simulink model "SCARA_Robot"  (R2018b)
settings: Solver=FixedStepAuto  StartTime=0.0  StopTime=5  FixedStep=0.001  MaxStep=0.001  MinStep=0.0001  RelTol=1e-3
model workspace: external: MATLAB File G:\MATLAB\SCARA\SCARA_Robot_DataFile.m (data not in the file)
values from neighbouring files (symbols this model uses):
  Ball = struct    [SCARA_Robot_DataFile.m]
  Plane = struct    [SCARA_Robot_DataFile.m]
  smiData = struct    [SCARA_Robot_DataFile.m]
undefined symbols (not defined in the file or in its folder): sigbuilder_block, X, Y, Z
libraries: sm_lib x160, nesl_utility x83, robotmaniplib x17, Contact_Forces_Lib x6, Parts_Lib x4, simulink x1
(part 1 of 4)
settings Model: Creator=wqq  LastModifiedBy=wqq
settings SolverCC: InitialStep=0.0001

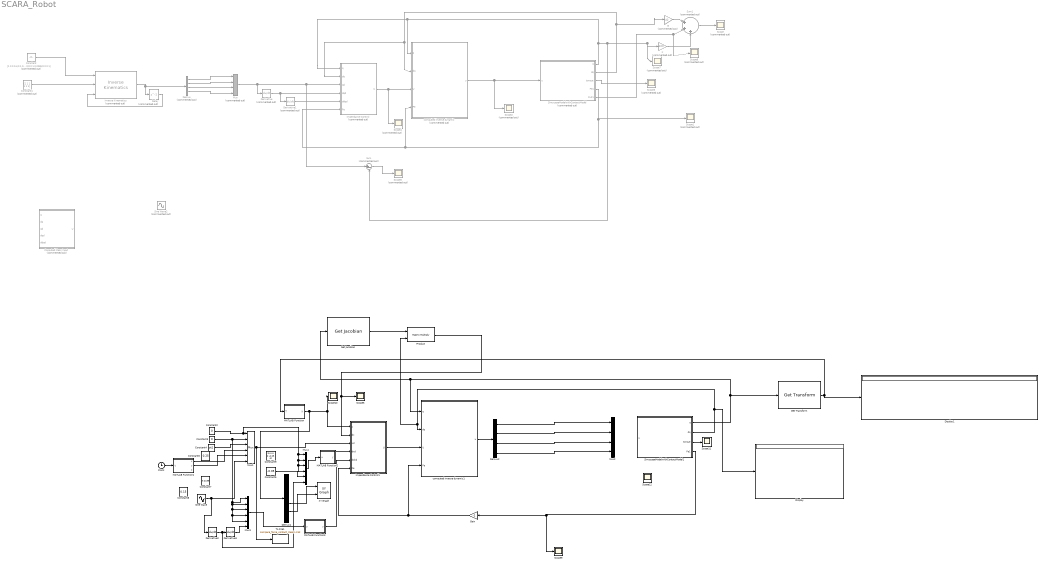
== system SCARA_Robot ==
  B : Gain  Commented=on  Gain=40
  Clock : Clock
  Conputed Mass Input : Subsystem  Commented=on
  Constant : Constant  Commented=on  Value=[1 0 0 0.4;0 1 0 0;0 0 1 0.2235;0 0 0 1]  VectorParams1D=off
  Constant1 : Constant  Commented=on  Value=[1 1 1 1 1 1]
  Constant2 : Constant  Value=0
  Constant3 : Constant  Value=0
  Constant4 : Constant  Value=pi/2
  Constant5 : Constant  Value=-0.05  VectorParams1D=off
  Constant6 : Constant  Value=0.25
  Constant7 : Constant  Value=0.2235
  Constant8 : Constant  Value=0.15
  Constant9 : Constant  Value=[0 0 0 0 -0.05 0]  VectorParams1D=off
  Delay : Delay  Commented=on  DelayLength=1  InitialCondition=[0;0;0;0]
  Demux : Demux  Commented=on
  Demux1 : Demux  Outputs=6
  Demux2 : Demux
  Derivative : Derivative  Commented=on
  Derivative1 : Derivative  Commented=on
  Derivative2 : Derivative
  Derivative3 : Derivative
  Display : Display
  Display1 : Display
  Gain : Gain  Gain=-1
  Get Jacobian : robotmaniplib/Get Jacobian  RigidBodyTree=SCARA_Robot  EndEffector=Body5
      settings: SourceProductName=Robotics System Toolbox
  Get Transform : robotmaniplib/Get Transform  RigidBodyTree=SCARA_Robot  SourceBody=Body5  TargetBody=Body7
      settings: SourceProductName=Robotics System Toolbox
  Impendance Control : Subsystem  Commented=on
  Impendance Control1 : Subsystem
  Inverse Kinematics : robotmaniplib/Inverse Kinematics  Commented=on  RigidBodyTree=SCARA_Robot  EndEffector=Body5  ShowInfo=off  SolverName=BFGS Gradient Projection  EnforceJointLimits=on  MaxIterations=1500  MaxTime=10  GradientTolerance=1e-7  SolutionTolerance=1e-6  StepTolerance=1e-14  ErrorChangeTolerance=1e-12  UseErrorDamping=on  DampingBias=0.0025
      settings: SourceProductName=Robotics System Toolbox
  K : Gain  Commented=on  Gain=400
  MATLAB Function : MATLAB Function  TreatAsAtomicUnit=on
  MATLAB Function1 : MATLAB Function  TreatAsAtomicUnit=on
  MATLAB Function2 : MATLAB Function  TreatAsAtomicUnit=on
  MATLAB Function3 : MATLAB Function  TreatAsAtomicUnit=on
  Mux : Mux  Commented=on
  Mux1 : Mux  Inputs=6
  Mux2 : Mux
  Mux3 : Mux  Inputs=6
  Mux4 : Mux  Inputs=6
  Product : Product  Multiplication=Matrix(*)
  Scope{,1..4,6..8} (8 alike) : Scope  Commented=on
  Scope{5,9..12} (5 alike) : Scope
  SimscapeModelwithContactModel : Subsystem  Commented=on
  SimscapeModelwithContactModel1 : Subsystem
  Sine Wave : Sin  Amplitude=0.5  Bias=0.2235  Frequency=3  SampleTime=0
  Sine Wave2 : Sin  Commented=on  Amplitude=0.5  SampleTime=0
  Sum : Sum  Commented=on  Inputs=|+-
  Sum1 : Sum  Commented=on  Inputs=|+++
  To File1 : ToFile  Filename=compare_force_contact_RealX.mat  MatrixName=RealX  SaveFormat=Timeseries
  XY Graph : simulink/Sinks/XY Graph  xmin=-0.4  xmax=0.4  ymin=-0.4  ymax=0.4  st=-1
  computed Inverse dynamic : Subsystem  Commented=on
  computed Inverse dynamic1 : Subsystem
  wires:
  computed Inverse dynamic/1(u) -> SimscapeModelwithContactModel/1(u), Scope2/1
  SimscapeModelwithContactModel/1(q) -> Scope7/1, K/1, Sum/2, computed Inverse dynamic/1(q), Impendance Control/1(q)
  SimscapeModelwithContactModel/3(torque) -> Scope3/1
  Impendance Control/1(U) -> Scope4/1, computed Inverse dynamic/3(U)
  Mux/1 -> Derivative/1, Sum/1, Impendance Control/3(qd)
  Derivative/1 -> Derivative1/1, Impendance Control/4(dqd)
  Derivative1/1 -> Impendance Control/5(ddqd)
  SimscapeModelwithContactModel/4(Fe1) -> Impendance Control/6(Fe), computed Inverse dynamic/4(Fe), Scope1/1
  Sum/1 -> Scope6/1
  SimscapeModelwithContactModel/2(dq) -> B/1, computed Inverse dynamic/2(dq), Impendance Control/2(dq)
  Sum1/1 -> Scope/1
  K/1 -> Sum1/3
  B/1 -> Sum1/1
  SimscapeModelwithContactModel/5(Out1) -> Scope8/1, Sum1/2
  Impendance Control1/1(U) -> computed Inverse dynamic1/3(U)
  SimscapeModelwithContactModel1/2(dq) -> Display/1, computed Inverse dynamic1/2(dq), Product/2
  SimscapeModelwithContactModel1/4(Fe1) -> Scope9/1, Gain/1
  Get Transform/1 -> MATLAB Function/1(T), Display1/1
  MATLAB Function/1(X) -> Demux1/1, Scope10/1, Impendance Control1/1(x)
  Inverse Kinematics/1 -> Demux/1, Delay/1
  Delay/1 -> Inverse Kinematics/3
  Constant/1 -> Inverse Kinematics/1
  Constant1/1 -> Inverse Kinematics/2
  Demux/1 -> Mux/1
  Demux/2 -> Mux/2
  Demux/3 -> Mux/3
  Demux/4 -> Mux/4
  Constant2/1 -> Mux4/1, Mux4/2, Mux4/3, Mux4/4, Mux1/1
  Constant3/1 -> Mux3/1, Mux3/2, Mux3/3, Mux3/4, Mux3/5, Mux1/2
  Constant4/1 -> Mux1/3
  Clock/1 -> MATLAB Function1/1(t)
  Get Jacobian/1 -> Product/1
  Product/1 -> Impendance Control1/2(dx), Scope5/1
  Demux1/4 -> XY Graph/1
  Demux1/5 -> XY Graph/2
  SimscapeModelwithContactModel1/1(q) -> Get Transform/1, computed Inverse dynamic1/1(q), Get Jacobian/1
  SimscapeModelwithContactModel1/3(torque) -> Scope11/1
  Gain/1 -> computed Inverse dynamic1/4(Fe), Impendance Control1/6(Fe)
  computed Inverse dynamic1/1(u) -> Demux2/1
  Sine Wave/1 -> Derivative2/1, Mux1/6
  Mux1/1 -> To File1/1, Impendance Control1/3(xd)
  Demux2/2 -> Mux2/2
  Demux2/3 -> Mux2/3
  Demux2/4 -> Mux2/4
  Demux2/1 -> Mux2/1
  MATLAB Function1/1(x) -> Mux1/4
  MATLAB Function1/2(y) -> Mux1/5
  Derivative2/1 -> Mux4/6, Derivative3/1
  Derivative3/1 -> Mux3/6
  Constant5/1 -> Mux4/5
  Mux4/1 -> MATLAB Function2/1(u)
  Mux3/1 -> MATLAB Function3/1(u)
  MATLAB Function3/1(y) -> Impendance Control1/5(ddxd)
  MATLAB Function2/1(y) -> Impendance Control1/4(dxd)

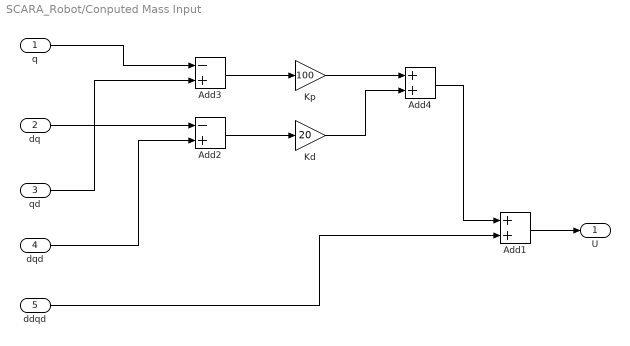
== system SCARA_Robot/Conputed Mass Input ==
  q : Inport
  dq : Inport  Port=2
  qd : Inport  Port=3
  dqd : Inport  Port=4
  ddqd : Inport  Port=5
  Add1 : Sum
  Add2 : Sum  Inputs=-+
  Add3 : Sum  Inputs=-+
  Add4 : Sum
  Kd : Gain  Gain=20
  Kp : Gain  Gain=100
  U : Outport
  wires:
  Add4/1 -> Add1/1
  Add2/1 -> Kd/1
  Kp/1 -> Add4/1
  Add3/1 -> Kp/1
  q/1 -> Add3/1
  dq/1 -> Add2/1
  dqd/1 -> Add2/2
  Add1/1 -> U/1
  Kd/1 -> Add4/2
  qd/1 -> Add3/2
  ddqd/1 -> Add1/2

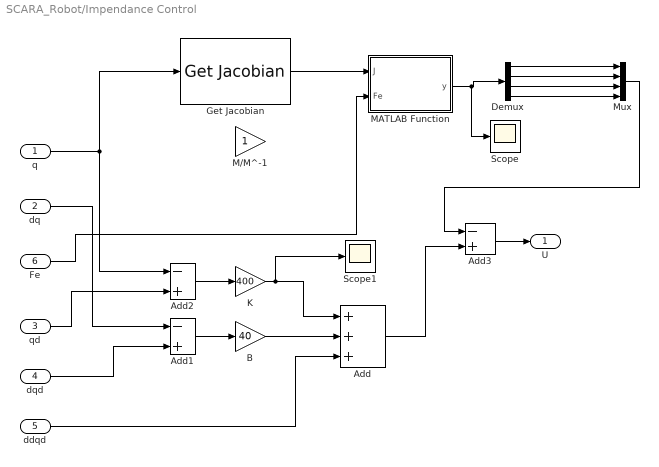
== system SCARA_Robot/Impendance Control ==
  q : Inport
  dq : Inport  Port=2
  qd : Inport  Port=3
  dqd : Inport  Port=4
  ddqd : Inport  Port=5
  Fe : Inport  Port=6
  Add : Sum  Inputs=+++
  Add1 : Sum  Inputs=-+
  Add2 : Sum  Inputs=-+
  Add3 : Sum  Inputs=-+
  B : Gain  Gain=40
  Demux : Demux
  Get Jacobian : robotmaniplib/Get Jacobian  RigidBodyTree=SCARA_Robot  EndEffector=Body5
      settings: SourceProductName=Robotics System Toolbox
  K : Gain  Gain=400
  M/M^-1 : Gain
  MATLAB Function : MATLAB Function  TreatAsAtomicUnit=on
  Mux : Mux
  Scope : Scope
  Scope1 : Scope
  U : Outport
  wires:
  ddqd/1 -> Add/3
  dqd/1 -> Add1/2
  dq/1 -> Add1/1
  Add1/1 -> B/1
  B/1 -> Add/2
  qd/1 -> Add2/2
  Add2/1 -> K/1
  K/1 -> Scope1/1, Add/1
  Add/1 -> Add3/2
  Add3/1 -> U/1
  q/1 -> Add2/1, Get Jacobian/1
  Get Jacobian/1 -> MATLAB Function/1(J)
  Fe/1 -> MATLAB Function/2(Fe)
  MATLAB Function/1(y) -> Scope/1, Demux/1
  Demux/1 -> Mux/1
  Demux/2 -> Mux/2
  Demux/3 -> Mux/3
  Demux/4 -> Mux/4
  Mux/1 -> Add3/1

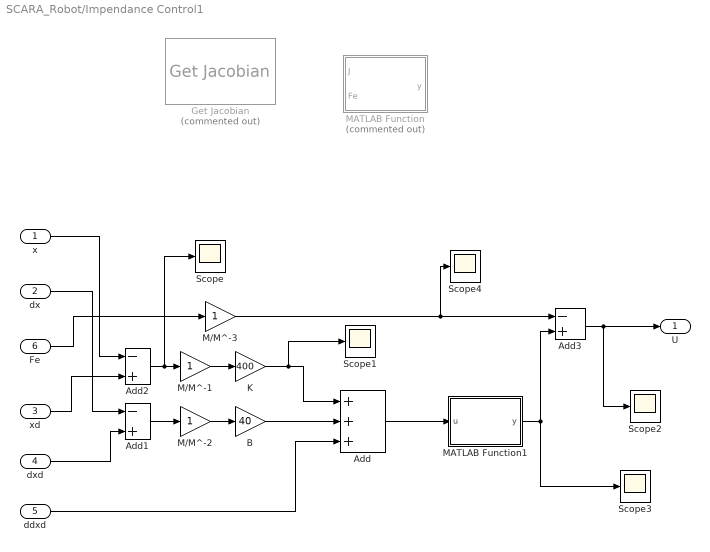
== system SCARA_Robot/Impendance Control1 ==
  x : Inport
  dx : Inport  Port=2
  xd : Inport  Port=3
  dxd : Inport  Port=4
  ddxd : Inport  Port=5
  Fe : Inport  Port=6
  Add : Sum  Inputs=+++
  Add1 : Sum  Inputs=-+
  Add2 : Sum  Inputs=-+
  Add3 : Sum  Inputs=-+
  B : Gain  Gain=40
  Get Jacobian : robotmaniplib/Get Jacobian  Commented=on  RigidBodyTree=SCARA_Robot  EndEffector=Body5
      settings: SourceProductName=Robotics System Toolbox
  K : Gain  Gain=400
  M/M^-1 : Gain
  M/M^-2 : Gain
  M/M^-3 : Gain
  MATLAB Function : MATLAB Function  Commented=on  TreatAsAtomicUnit=on
  MATLAB Function1 : MATLAB Function  TreatAsAtomicUnit=on
  Scope{,1..4} (5 alike) : Scope
  U : Outport
  wires:
  ddxd/1 -> Add/3
  dxd/1 -> Add1/2
  dx/1 -> Add1/1
  Add1/1 -> M/M^-2/1
  B/1 -> Add/2
  xd/1 -> Add2/2
  Add2/1 -> Scope/1, M/M^-1/1
  K/1 -> Scope1/1, Add/1
  Add/1 -> MATLAB Function1/1(u)
  x/1 -> Add2/1
  Fe/1 -> M/M^-3/1
  M/M^-1/1 -> K/1
  M/M^-2/1 -> B/1
  M/M^-3/1 -> Scope4/1, Add3/1
  MATLAB Function1/1(y) -> Add3/2, Scope3/1
  Add3/1 -> Scope2/1, U/1

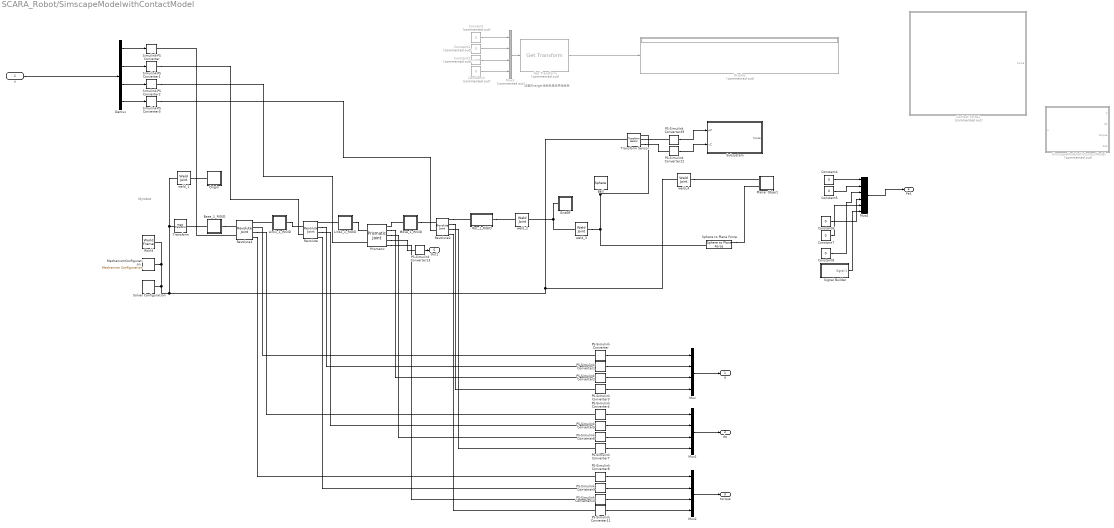
== system SCARA_Robot/SimscapeModelwithContactModel ==
  note: 这里的target坐标系是世界坐标系
  note: Myrobot
  u : Inport
  Ball : Parts_Lib/Sphere  Tag=CustomStyle  sph_radius=Ball.radius  sph_density=Ball.density  sph_color=red  sph_opacity=1  mark_type=Rings on center planes  arc_width=[40 50]  arc_angle=60  ring_width=5  ring_irad=0.95  mark_color=axes  mark_opacity_x=1  mark_opacity_y=1  mark_opacity_z=1  mark_opacity=1  ring_opacity=0  arc_opacity=0  arc_extr_data=0
  Base_1_RIGID : Subsystem
  Constant : Constant  Commented=on  Value=0
  Constant1 : Constant  Commented=on  Value=0
  Constant2 : Constant  Commented=on  Value=-0.2235
  Constant3 : Constant  Commented=on  Value=0
  Constant{4..8} (5 alike) : Constant  Value=0
  Contact Force1 : Subsystem  Commented=on
  Demux : Demux
  Display : Display  Commented=on
  EndEff : Subsystem
  Get Transform : robotmaniplib/Get Transform  Commented=on  RigidBodyTree=SCARA_Robot  SourceBody=Body5  TargetBody=Body7
      settings: SourceProductName=Robotics System Toolbox
  Link1_1_RIGID : Subsystem
  Link2_1_RIGID : Subsystem
  MechanismConfiguration : sm_lib/Utilities/Mechanism Configuration  UniformGravity=Constant  GravityVector=[0 0 -9.80665]  GravityUnits=m/s^2  LinearizationDelta=0.001
  Move_1_RIGID : Subsystem
  Mux : Mux
  Mux1 : Mux
  Mux2 : Mux
  Mux3 : Mux  Commented=on
  Mux4 : Mux  Inputs=6
  Origin : Subsystem
  PS-Simulink Converter{,1..13,29} (15 alike) : nesl_utility/PS-Simulink Converter  PhysicalDomain=network_engine_domain  SubClassName=ps_output  LeftPortType=input  RightPortType=output  PseudoPeriodic=off  Frequencies=[]  Unit=1  AffineConversion=off
  Planar Object : Subsystem
  Prismatic : sm_lib/Joints/Prismatic Joint  SenseConstraintForce=off  SenseConstraintForceX=off  SenseConstraintForceY=off  SenseConstraintForceZ=off  SenseConstraintTorque=off  SenseConstraintTorqueX=off  SenseConstraintTorqueY=off  SenseConstraintTorqueZ=off  SenseTotalForce=off  SenseTotalForceX=off  SenseTotalForceY=off  SenseTotalForceZ=off  SenseTotalTorque=off  SenseTotalTorqueX=off  SenseTotalTorqueY=off  SenseTotalTorqueZ=off  CompositeWrenchDir=FollowerOnBase  CompositeWrenchFrame=BaseFrame  EquilibriumPosition=0  EquilibriumPositionUnits=m  SpringStiffness=0  SpringStiffnessUnits=N/m  DampingCoefficient=0  DampingCoefficientUnits=N/(m/s)  TorqueActuationMode=InputTorque  MotionActuationMode=ComputedMotion  SensePosition=on  SenseVelocity=on  SenseAcceleration=on  SenseTorqueForce=on  PositionTargetSpecify=on  PositionTargetPriority=High  PositionTargetValue=smiData.PrismaticJoint(1).Pz.Pos  PositionTargetValueUnits=m  VelocityTargetSpecify=off  VelocityTargetPriority=High  VelocityTargetValue=0  VelocityTargetValueUnits=m/s
  Revolute : sm_lib/Joints/Revolute Joint  SenseConstraintForce=off  SenseConstraintForceX=off  SenseConstraintForceY=off  SenseConstraintForceZ=off  SenseConstraintTorque=off  SenseConstraintTorqueX=off  SenseConstraintTorqueY=off  SenseConstraintTorqueZ=off  SenseTotalForce=off  SenseTotalForceX=off  SenseTotalForceY=off  SenseTotalForceZ=off  SenseTotalTorque=off  SenseTotalTorqueX=off  SenseTotalTorqueY=off  SenseTotalTorqueZ=off  CompositeWrenchDir=FollowerOnBase  CompositeWrenchFrame=BaseFrame  EquilibriumPosition=0  EquilibriumPositionUnits=rad  SpringStiffness=0  SpringStiffnessUnits=N*m/rad  DampingCoefficient=0  DampingCoefficientUnits=N*m/(rad/s)  TorqueActuationMode=InputTorque  MotionActuationMode=ComputedMotion  SensePosition=on  SenseVelocity=on  SenseAcceleration=off  SenseTorqueForce=on  PositionTargetSpecify=on  PositionTargetPriority=High  PositionTargetValue=smiData.RevoluteJoint(1).Rz.Pos  PositionTargetValueUnits=deg  VelocityTargetSpecify=off  VelocityTargetPriority=High  VelocityTargetValue=0  VelocityTargetValueUnits=deg/s
  Revolute1 : sm_lib/Joints/Revolute Joint  SenseConstraintForce=off  SenseConstraintForceX=off  SenseConstraintForceY=off  SenseConstraintForceZ=off  SenseConstraintTorque=off  SenseConstraintTorqueX=off  SenseConstraintTorqueY=off  SenseConstraintTorqueZ=off  SenseTotalForce=off  SenseTotalForceX=off  SenseTotalForceY=off  SenseTotalForceZ=off  SenseTotalTorque=off  SenseTotalTorqueX=off  SenseTotalTorqueY=off  SenseTotalTorqueZ=off  CompositeWrenchDir=FollowerOnBase  CompositeWrenchFrame=BaseFrame  EquilibriumPosition=0  EquilibriumPositionUnits=rad  SpringStiffness=0  SpringStiffnessUnits=N*m/rad  DampingCoefficient=0  DampingCoefficientUnits=N*m/(rad/s)  TorqueActuationMode=InputTorque  MotionActuationMode=ComputedMotion  SensePosition=on  SenseVelocity=on  SenseAcceleration=off  SenseTorqueForce=on  PositionTargetSpecify=on  PositionTargetPriority=High  PositionTargetValue=smiData.RevoluteJoint(2).Rz.Pos  PositionTargetValueUnits=deg  VelocityTargetSpecify=off  VelocityTargetPriority=High  VelocityTargetValue=0  VelocityTargetValueUnits=deg/s
  Revolute2 : sm_lib/Joints/Revolute Joint  SenseConstraintForce=off  SenseConstraintForceX=off  SenseConstraintForceY=off  SenseConstraintForceZ=off  SenseConstraintTorque=off  SenseConstraintTorqueX=off  SenseConstraintTorqueY=off  SenseConstraintTorqueZ=off  SenseTotalForce=off  SenseTotalForceX=off  SenseTotalForceY=off  SenseTotalForceZ=off  SenseTotalTorque=off  SenseTotalTorqueX=off  SenseTotalTorqueY=off  SenseTotalTorqueZ=off  CompositeWrenchDir=FollowerOnBase  CompositeWrenchFrame=BaseFrame  EquilibriumPosition=0  EquilibriumPositionUnits=rad  SpringStiffness=0  SpringStiffnessUnits=N*m/rad  DampingCoefficient=0  DampingCoefficientUnits=N*m/(rad/s)  TorqueActuationMode=InputTorque  MotionActuationMode=ComputedMotion  SensePosition=on  SenseVelocity=on  SenseAcceleration=off  SenseTorqueForce=on  PositionTargetSpecify=on  PositionTargetPriority=High  PositionTargetValue=smiData.RevoluteJoint(3).Rz.Pos  PositionTargetValueUnits=deg  VelocityTargetSpecify=off  VelocityTargetPriority=High  VelocityTargetValue=0  VelocityTargetValueUnits=deg/s
  Rot_1_RIGID : Subsystem
  Signal Builder : Subsystem  Tag=STV Subsys  LoadFcn=sigbuilder_block('load');  StartFcn=sigbuilder_block('start');  StopFcn=sigbuilder_block('stop');  ClipboardFcn=sigbuilder_block('clipboard');  mask(Sigbuilder block){tuvar=[0:10]}
      mask help: Simulink:masks:SigbuilderBlock_MD
      mask init:
      | if ~strcmp(get_param(bdroot(gcbh),'SimulationStatus'),'stopped') tuvar = sigbuilder_block('maskInit'); end
      settings: CopyFcn=sigbuilder_block('copy');  DeleteFcn=sigbuilder_block('delete');  ModelCloseFcn=sigbuilder_block('modelClose');  PreSaveFcn=sigbuilder_block('preSave');  PauseFcn=sigbuilder_block('pause');  ContinueFcn=sigbuilder_block('continue');  NameChangeFcn=sigbuilder_block('namechange');  OpenFcn=sigbuilder_block('open',[437.6 199.2 550.4 400 ]);  CloseFcn=sigbuilder_block('close');
      mask Display: plot(0, 0, 100, 100,[2, 2, 32, 32, 2], [68, 8, 8, 68, 68],[32, 2], [38, 38], [32, 19, 2],[53, 60, 44], [32, 17, 17, 2],[16, 16, 31, 31]);txt = getActiveGroup(gcbh);text(2, 100, txt,'verticalAlignment', 'top');
  SimscapeModelwithContactModel : Subsystem  Commented=on
  Simulink-PS Converter{,1..3} (4 alike) : nesl_utility/Simulink-PS Converter  PhysicalDomain=network_engine_domain  SubClassName=ps_input  LeftPortType=input  RightPortType=output  PseudoPeriodic=off  Frequencies=[]  NoiseDistribution=none  NoiseParameters=[]  Unit=1  AffineConversion=off  FilteringAndDerivatives=provide  SimscapeFilterOrder=1  InputFilterTimeConstant=0.001  UdotUserProvided=0
  Solver Configuration : nesl_utility/Solver Configuration  PhysicalDomain=network_engine_domain  SubClassName=solver  LeftPortType=input  RightPortType=generic  Tones=[]  Harmonics=[]  SimulateNoise=off  Profile=off  UseLocalSampling=off  EnableSwitchedLinearOptims=on  FrequencyDomain=off  UseCCode=off  RelTol=0.001  AbsTol=1e-06  MinStep=1e-09  ToWorkspace=off  RevertToSquareIcSolve=off  NumHomotopyIterations=100  PhasorMode=off  PhasorModeNumHarmonics=1  DoDC=off  ResidualTolerance=1e-09  UseLocalSolver=off  LocalSolverChoice=NE_BACKWARD_EULER_ADVANCER  LocalSolverSampleTime=0.001  DoFixedCost=off  MaxNonlinIter=3  MaxModeIter=2  LinearAlgebra=auto  EquationFormulation=NE_TIME_EF  DelaysMemoryBudget=1024  AutomaticFiltering=on  FilteringTimeConstant=0.001  PartitionStorageMethod=AS_NEEDED  PartitionMemoryBudget=1024
  Sphere to Plane Force : Contact_Forces_Lib/3D/Sphere to Plane Force  sphere_rad=0.03  plane_lenx=1  plane_leny=1  plane_depth=0.1/2  force_law=Linear  k_contact=1e4  b_contact=1e2  pen_full_damp_F=1e-4  pen_exponent=1  custom_param_1=1  custom_param_2=1  friction_law=Stick-Slip Continuous  mu_kinetic=0.5  mu_static=0.7  v_thr=0.001  vis_on=off  vis_opc_en=0  vis_len_plaBz=0.005  vis_clr=[0.9 0.2 0.2]  vis_opc=0.7
  Subsystem : Subsystem
  Transform : sm_lib/Frames and Transforms/Rigid Transform  TranslationMethod=Cartesian  TranslationStandardOffset=0  TranslationLengthUnit=mm  TranslationStandardAxis=+Z  TranslationCartesianOffset=smiData.RigidTransform(9).translation  TranslationROffset=0  TranslationROffsetUnits=m  TranslationZOffset=0  TranslationZOffsetUnits=m  TranslationThetaOffset=0  TranslationThetaOffsetUnits=deg  RotationMethod=ArbitraryAxis  RotationAngleUnits=rad  RotationStandardAxis=+Z  RotationAngle=smiData.RigidTransform(9).angle  RotationArbitraryAxis=smiData.RigidTransform(9).axis  FollAlignAxisA=+X  BaseAlignAxisA=+Y  FollAlignAxisB=+Y  BaseAlignAxisB=+Z  RotationSequenceAxes=FollowerAxes  RotationSequence=XYX  RotationSequenceAngles=[0 0 0]  RotationSequenceAnglesUnits=deg  RotationMatrix=[1 0 0; 0 1 0; 0 0 1]
  Transform Sensor : sm_lib/Frames and Transforms/Transform Sensor  MeasurementFrame=World  SenseAngle=off  SenseAxis=off  SenseAngle1=off  SenseAngle2=off  SenseAngle3=off  SenseQ=off  SenseR=off  SenseOmegaX=off  SenseOmegaY=off  SenseOmegaZ=off  SenseOmega1=off  SenseOmega2=off  SenseOmega3=off  SenseQDot=off  SenseRDot=off  SenseAlphaX=off  SenseAlphaY=off  SenseAlphaZ=off  SenseAlpha1=off  SenseAlpha2=off  SenseAlpha3=off  SenseQDDot=off  SenseRDDot=off  SenseX=off  SenseY=off  SenseZ=on  SenseRad=off  SenseAzim=off  SenseDist=off  SenseInc=off  SenseXDot=off  SenseYDot=off  SenseZDot=on  SenseRadDot=off  SenseAzimDot=off  SenseDistDot=off  SenseIncDot=off  SenseXDDot=off  SenseYDDot=off  SenseZDDot=off  SenseRadDDot=off  SenseAzimDDot=off  SenseDistDDot=off  SenseIncDDot=off
  World : sm_lib/Frames and Transforms/World Frame
  weld_{1..4} (4 alike) : sm_lib/Joints/Weld Joint  SenseConstraintForce=off  SenseConstraintForceX=off  SenseConstraintForceY=off  SenseConstraintForceZ=off  SenseConstraintTorque=off  SenseConstraintTorqueX=off  SenseConstraintTorqueY=off  SenseConstraintTorqueZ=off  SenseTotalForce=off  SenseTotalForceX=off  SenseTotalForceY=off  SenseTotalForceZ=off  SenseTotalTorque=off  SenseTotalTorqueX=off  SenseTotalTorqueY=off  SenseTotalTorqueZ=off  CompositeWrenchDir=FollowerOnBase  CompositeWrenchFrame=BaseFrame
  q : Outport
  dq : Outport  Port=2
  torque : Outport  Port=3
  Fe1 : Outport  Port=4
  Out1 : Outport  Port=5
  wires:
  Demux/4 -> Simulink-PS Converter3/1
  Mux1/1 -> dq/1
  PS-Simulink Converter10/1 -> Mux2/3
  PS-Simulink Converter8/1 -> Mux2/1
  Demux/3 -> Simulink-PS Converter2/1
  Demux/1 -> Simulink-PS Converter/1
  PS-Simulink Converter11/1 -> Mux2/4
  PS-Simulink Converter5/1 -> Mux1/2
  PS-Simulink Converter/1 -> Mux/1
  Mux2/1 -> torque/1
  PS-Simulink Converter1/1 -> Mux/2
  Demux/2 -> Simulink-PS Converter1/1
  PS-Simulink Converter9/1 -> Mux2/2
  PS-Simulink Converter6/1 -> Mux1/3
  PS-Simulink Converter7/1 -> Mux1/4
  PS-Simulink Converter4/1 -> Mux1/1
  Mux/1 -> q/1
  PS-Simulink Converter2/1 -> Mux/3
  PS-Simulink Converter3/1 -> Mux/4
  Mux3/1 -> Get Transform/1
  Constant/1 -> Mux3/1
  Constant1/1 -> Mux3/2
  Constant2/1 -> Mux3/3
  Constant3/1 -> Mux3/4
  u/1 -> Demux/1
  Get Transform/1 -> Display/1
  Constant4/1 -> Mux4/1
  Constant5/1 -> Mux4/2
  Mux4/1 -> Fe1/1
  Constant7/1 -> Mux4/5
  Constant8/1 -> Mux4/3
  Constant6/1 -> Mux4/4
  PS-Simulink Converter29/1 -> Subsystem/1(pZ)
  PS-Simulink Converter12/1 -> Subsystem/2(vZ)
  Signal Builder/1(Signal 1) -> Mux4/6
  PS-Simulink Converter13/1 -> Out1/1
  connections:
  Revolute2/RConn3 -- PS-Simulink Converter7/LConn1
  Revolute/RConn2 -- PS-Simulink Converter1/LConn1
  Link2_1_RIGID/LConn1 -- Revolute/RConn1
  Move_1_RIGID/LConn1 -- Prismatic/RConn1
  Link1_1_RIGID/LConn1 -- Revolute1/RConn1
  Base_1_RIGID/LConn1 -- Transform/RConn1
  Revolute2/RConn2 -- PS-Simulink Converter3/LConn1
  Revolute1/LConn2 -- Simulink-PS Converter/RConn1
  Revolute1/RConn3 -- PS-Simulink Converter4/LConn1
  Simulink-PS Converter3/RConn1 -- Revolute2/LConn2
  Revolute1/RConn4 -- PS-Simulink Converter8/LConn1
  Move_1_RIGID/RConn1 -- Revolute2/LConn1
  PS-Simulink Converter/LConn1 -- Revolute1/RConn2
  Revolute/RConn4 -- PS-Simulink Converter9/LConn1
  Link2_1_RIGID/RConn1 -- Prismatic/LConn1
  Base_1_RIGID/RConn1 -- Revolute1/LConn1
  Link1_1_RIGID/RConn1 -- Revolute/LConn1
  Revolute2/RConn1 -- Rot_1_RIGID/LConn1
  Prismatic/RConn2 -- PS-Simulink Converter2/LConn1
  Revolute2/RConn4 -- PS-Simulink Converter11/LConn1
  Simulink-PS Converter2/RConn1 -- Prismatic/LConn2
  Simulink-PS Converter1/RConn1 -- Revolute/LConn2
  Revolute/RConn3 -- PS-Simulink Converter5/LConn1
  Prismatic/RConn3 -- PS-Simulink Converter6/LConn1
  Rot_1_RIGID/RConn1 -- weld_2/LConn1
  EndEff/LConn1 -- weld_3/LConn1 -- weld_2/RConn1
  Origin/LConn1 -- weld_1/RConn1
  Ball/LConn1 -- Sphere to Plane Force/LConn1 -- weld_3/RConn1 -- Transform Sensor/RConn1
  weld_1/LConn1 -- weld_4/LConn1 -- Transform Sensor/LConn1 -- World/RConn1 -- MechanismConfiguration/RConn1 -- Solver Configuration/RConn1 -- Transform/LConn1
  PS-Simulink Converter29/LConn1 -- Transform Sensor/RConn2
  Transform Sensor/RConn3 -- PS-Simulink Converter12/LConn1
  weld_4/RConn1 -- Planar Object/LConn1
  Prismatic/RConn4 -- PS-Simulink Converter13/LConn1
  Prismatic/RConn5 -- PS-Simulink Converter10/LConn1
  Sphere to Plane Force/RConn1 -- Planar Object/LConn2

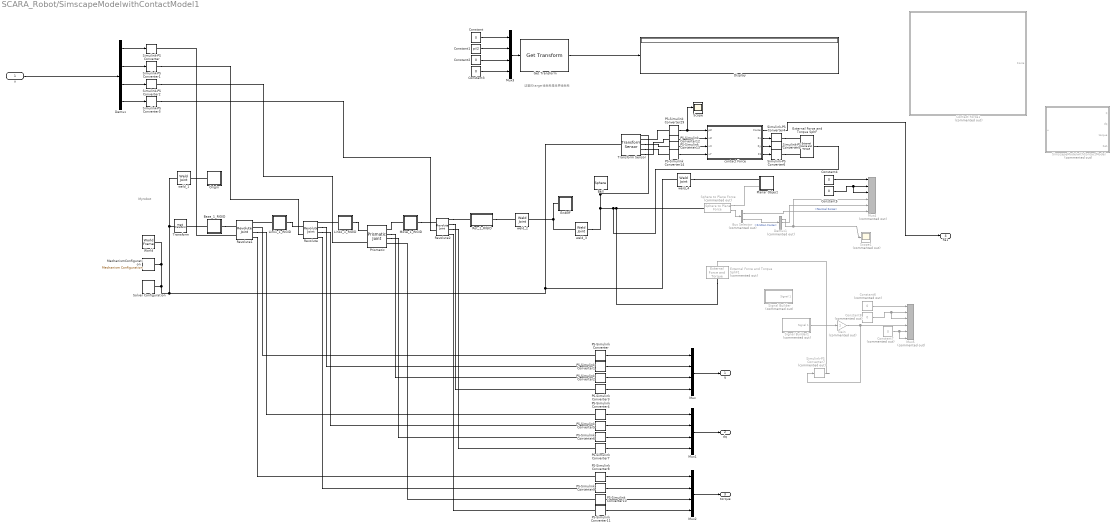
== system SCARA_Robot/SimscapeModelwithContactModel1 ==
  note: 这里的target坐标系是世界坐标系
  note: Myrobot
  u : Inport
  Ball : Parts_Lib/Sphere  Tag=CustomStyle  sph_radius=Ball.radius  sph_density=Ball.density  sph_color=red  sph_opacity=1  mark_type=Rings on center planes  arc_width=[40 50]  arc_angle=60  ring_width=5  ring_irad=0.95  mark_color=axes  mark_opacity_x=1  mark_opacity_y=1  mark_opacity_z=1  mark_opacity=1  ring_opacity=0  arc_opacity=0  arc_extr_data=0
  Base_1_RIGID : Subsystem
  Bus Selector : BusSelector  Commented=on  OutputSignals=Normal Force,Friction Force
  Constant{,2..5} (5 alike) : Constant  Value=0
  Constant1 : Constant  Value=pi/2
  Constant6 : Constant  Commented=on  Value=0
  Constant7 : Constant  Commented=on  Value=0
  Constant8 : Constant  Commented=on  Value=0
  Contact Force1 : Subsystem  Commented=on
  Demux : Demux
  Demux1 : Demux  Commented=on  Outputs=3
  Display : Display
  EndEff : Subsystem
  External Force and Torque SphF : sm_lib/Forces and Torques/External Force and Torque  ForceResolutionFrame=AttachedFrame  EnableForceX=on  EnableForceY=on  EnableForceZ=on  EnableForce=off  TorqueResolutionFrame=AttachedFrame  EnableTorqueX=off  EnableTorqueY=off  EnableTorqueZ=off  EnableTorque=off
  External Force and Torque SphF1 : sm_lib/Forces and Torques/External Force and Torque  Commented=on  ForceResolutionFrame=World  EnableForceX=on  EnableForceY=off  EnableForceZ=off  EnableForce=off  TorqueResolutionFrame=AttachedFrame  EnableTorqueX=off  EnableTorqueY=off  EnableTorqueZ=off  EnableTorque=off
  Gain : Gain  Commented=on
  Get Transform : robotmaniplib/Get Transform  RigidBodyTree=SCARA_Robot  SourceBody=Body5  TargetBody=Body7
      settings: SourceProductName=Robotics System Toolbox
  Link1_1_RIGID : Subsystem
  Link2_1_RIGID : Subsystem
  MechanismConfiguration : sm_lib/Utilities/Mechanism Configuration  UniformGravity=Constant  GravityVector=[0 0 -9.80665]  GravityUnits=m/s^2  LinearizationDelta=0.001
  Move_1_RIGID : Subsystem
  Mux{,1..3} (4 alike) : Mux
  Mux4 : Mux  Commented=on  Inputs=6
  Mux5 : Mux  Commented=on  Inputs=6
  Origin : Subsystem
  PS-Simulink Converter{,1..14,29} (16 alike) : nesl_utility/PS-Simulink Converter  PhysicalDomain=network_engine_domain  SubClassName=ps_output  LeftPortType=input  RightPortType=output  PseudoPeriodic=off  Frequencies=[]  Unit=1  AffineConversion=off
  Planar Object : Subsystem
  Prismatic : sm_lib/Joints/Prismatic Joint  SenseConstraintForce=off  SenseConstraintForceX=off  SenseConstraintForceY=off  SenseConstraintForceZ=off  SenseConstraintTorque=off  SenseConstraintTorqueX=off  SenseConstraintTorqueY=off  SenseConstraintTorqueZ=off  SenseTotalForce=off  SenseTotalForceX=off  SenseTotalForceY=off  SenseTotalForceZ=off  SenseTotalTorque=off  SenseTotalTorqueX=off  SenseTotalTorqueY=off  SenseTotalTorqueZ=off  CompositeWrenchDir=FollowerOnBase  CompositeWrenchFrame=BaseFrame  EquilibriumPosition=0  EquilibriumPositionUnits=m  SpringStiffness=0  SpringStiffnessUnits=N/m  DampingCoefficient=0  DampingCoefficientUnits=N/(m/s)  TorqueActuationMode=InputTorque  MotionActuationMode=ComputedMotion  SensePosition=on  SenseVelocity=on  SenseAcceleration=off  SenseTorqueForce=on  PositionTargetSpecify=on  PositionTargetPriority=High  PositionTargetValue=smiData.PrismaticJoint(1).Pz.Pos  PositionTargetValueUnits=m  VelocityTargetSpecify=off  VelocityTargetPriority=High  VelocityTargetValue=0  VelocityTargetValueUnits=m/s
  Revolute : sm_lib/Joints/Revolute Joint  SenseConstraintForce=off  SenseConstraintForceX=off  SenseConstraintForceY=off  SenseConstraintForceZ=off  SenseConstraintTorque=off  SenseConstraintTorqueX=off  SenseConstraintTorqueY=off  SenseConstraintTorqueZ=off  SenseTotalForce=off  SenseTotalForceX=off  SenseTotalForceY=off  SenseTotalForceZ=off  SenseTotalTorque=off  SenseTotalTorqueX=off  SenseTotalTorqueY=off  SenseTotalTorqueZ=off  CompositeWrenchDir=FollowerOnBase  CompositeWrenchFrame=BaseFrame  EquilibriumPosition=0  EquilibriumPositionUnits=rad  SpringStiffness=0  SpringStiffnessUnits=N*m/rad  DampingCoefficient=0  DampingCoefficientUnits=N*m/(rad/s)  TorqueActuationMode=InputTorque  MotionActuationMode=ComputedMotion  SensePosition=on  SenseVelocity=on  SenseAcceleration=off  SenseTorqueForce=on  PositionTargetSpecify=on  PositionTargetPriority=High  PositionTargetValue=90  PositionTargetValueUnits=deg  VelocityTargetSpecify=off  VelocityTargetPriority=High  VelocityTargetValue=0  VelocityTargetValueUnits=deg/s
  Revolute1 : sm_lib/Joints/Revolute Joint  SenseConstraintForce=off  SenseConstraintForceX=off  SenseConstraintForceY=off  SenseConstraintForceZ=off  SenseConstraintTorque=off  SenseConstraintTorqueX=off  SenseConstraintTorqueY=off  SenseConstraintTorqueZ=off  SenseTotalForce=off  SenseTotalForceX=off  SenseTotalForceY=off  SenseTotalForceZ=off  SenseTotalTorque=off  SenseTotalTorqueX=off  SenseTotalTorqueY=off  SenseTotalTorqueZ=off  CompositeWrenchDir=FollowerOnBase  CompositeWrenchFrame=BaseFrame  EquilibriumPosition=0  EquilibriumPositionUnits=rad  SpringStiffness=0  SpringStiffnessUnits=N*m/rad  DampingCoefficient=0  DampingCoefficientUnits=N*m/(rad/s)  TorqueActuationMode=InputTorque  MotionActuationMode=ComputedMotion  SensePosition=on  SenseVelocity=on  SenseAcceleration=off  SenseTorqueForce=on  PositionTargetSpecify=on  PositionTargetPriority=High  PositionTargetValue=smiData.RevoluteJoint(2).Rz.Pos  PositionTargetValueUnits=deg  VelocityTargetSpecify=off  VelocityTargetPriority=High  VelocityTargetValue=0  VelocityTargetValueUnits=deg/s
  Revolute2 : sm_lib/Joints/Revolute Joint  SenseConstraintForce=off  SenseConstraintForceX=off  SenseConstraintForceY=off  SenseConstraintForceZ=off  SenseConstraintTorque=off  SenseConstraintTorqueX=off  SenseConstraintTorqueY=off  SenseConstraintTorqueZ=off  SenseTotalForce=off  SenseTotalForceX=off  SenseTotalForceY=off  SenseTotalForceZ=off  SenseTotalTorque=off  SenseTotalTorqueX=off  SenseTotalTorqueY=off  SenseTotalTorqueZ=off  CompositeWrenchDir=FollowerOnBase  CompositeWrenchFrame=BaseFrame  EquilibriumPosition=0  EquilibriumPositionUnits=rad  SpringStiffness=0  SpringStiffnessUnits=N*m/rad  DampingCoefficient=0  DampingCoefficientUnits=N*m/(rad/s)  TorqueActuationMode=InputTorque  MotionActuationMode=ComputedMotion  SensePosition=on  SenseVelocity=on  SenseAcceleration=off  SenseTorqueForce=on  PositionTargetSpecify=on  PositionTargetPriority=High  PositionTargetValue=smiData.RevoluteJoint(3).Rz.Pos  PositionTargetValueUnits=deg  VelocityTargetSpecify=off  VelocityTargetPriority=High  VelocityTargetValue=0  VelocityTargetValueUnits=deg/s
  Rot_1_RIGID : Subsystem
  Scope : Scope
  Scope1 : Scope  Commented=on
  Signal Builder : Subsystem  Tag=STV Subsys  Commented=on  LoadFcn=sigbuilder_block('load');  StartFcn=sigbuilder_block('start');  StopFcn=sigbuilder_block('stop');  ClipboardFcn=sigbuilder_block('clipboard');  mask(Sigbuilder block){tuvar=[0:10]}
      mask help: Simulink:masks:SigbuilderBlock_MD
      mask init:
      | if ~strcmp(get_param(bdroot(gcbh),'SimulationStatus'),'stopped') tuvar = sigbuilder_block('maskInit'); end
      settings: CopyFcn=sigbuilder_block('copy');  DeleteFcn=sigbuilder_block('delete');  ModelCloseFcn=sigbuilder_block('modelClose');  PreSaveFcn=sigbuilder_block('preSave');  PauseFcn=sigbuilder_block('pause');  ContinueFcn=sigbuilder_block('continue');  NameChangeFcn=sigbuilder_block('namechange');  OpenFcn=sigbuilder_block('open',[437.6 199.2 550.4 400 ]);  CloseFcn=sigbuilder_block('close');
      mask Display: plot(0, 0, 100, 100,[2, 2, 32, 32, 2], [68, 8, 8, 68, 68],[32, 2], [38, 38], [32, 19, 2],[53, 60, 44], [32, 17, 17, 2],[16, 16, 31, 31]);txt = getActiveGroup(gcbh);text(2, 100, txt,'verticalAlignment', 'top');
  Signal Builder1 : Subsystem  Tag=STV Subsys  Commented=on  LoadFcn=sigbuilder_block('load');  StartFcn=sigbuilder_block('start');  StopFcn=sigbuilder_block('stop');  ClipboardFcn=sigbuilder_block('clipboard');  mask(Sigbuilder block){tuvar=[0:10]}
      mask help: Simulink:masks:SigbuilderBlock_MD
      mask init:
      | if ~strcmp(get_param(bdroot(gcbh),'SimulationStatus'),'stopped') tuvar = sigbuilder_block('maskInit'); end
      settings: CopyFcn=sigbuilder_block('copy');  DeleteFcn=sigbuilder_block('delete');  ModelCloseFcn=sigbuilder_block('modelClose');  PreSaveFcn=sigbuilder_block('preSave');  PauseFcn=sigbuilder_block('pause');  ContinueFcn=sigbuilder_block('continue');  NameChangeFcn=sigbuilder_block('namechange');  OpenFcn=sigbuilder_block('open',[415.2 152.4 550.8 400.2 ]);  CloseFcn=sigbuilder_block('close');
      mask Display: plot(0, 0, 100, 100,[2, 2, 32, 32, 2], [68, 8, 8, 68, 68],[32, 2], [38, 38], [32, 19, 2],[53, 60, 44], [32, 17, 17, 2],[16, 16, 31, 31]);txt = getActiveGroup(gcbh);text(2, 100, txt,'verticalAlignment', 'top');
  SimscapeModelwithContactModel : Subsystem  Commented=on
  Simulink-PS Converter{,1..6} (7 alike) : nesl_utility/Simulink-PS Converter  PhysicalDomain=network_engine_domain  SubClassName=ps_input  LeftPortType=input  RightPortType=output  PseudoPeriodic=off  Frequencies=[]  NoiseDistribution=none  NoiseParameters=[]  Unit=1  AffineConversion=off  FilteringAndDerivatives=provide  SimscapeFilterOrder=1  InputFilterTimeConstant=0.001  UdotUserProvided=0
  Simulink-PS Converter7 : nesl_utility/Simulink-PS Converter  Commented=on  PhysicalDomain=network_engine_domain  SubClassName=ps_input  LeftPortType=input  RightPortType=output  PseudoPeriodic=off  Frequencies=[]  NoiseDistribution=none  NoiseParameters=[]  Unit=1  AffineConversion=off  FilteringAndDerivatives=provide  SimscapeFilterOrder=1  InputFilterTimeConstant=0.001  UdotUserProvided=0
  Solver Configuration : nesl_utility/Solver Configuration  PhysicalDomain=network_engine_domain  SubClassName=solver  LeftPortType=input  RightPortType=generic  Tones=[]  Harmonics=[]  SimulateNoise=off  Profile=off  UseLocalSampling=off  EnableSwitchedLinearOptims=on  FrequencyDomain=off  UseCCode=off  RelTol=0.001  AbsTol=1e-06  MinStep=1e-09  ToWorkspace=off  RevertToSquareIcSolve=off  NumHomotopyIterations=100  PhasorMode=off  PhasorModeNumHarmonics=1  DoDC=off  ResidualTolerance=1e-09  UseLocalSolver=off  LocalSolverChoice=NE_BACKWARD_EULER_ADVANCER  LocalSolverSampleTime=0.001  DoFixedCost=off  MaxNonlinIter=3  MaxModeIter=2  LinearAlgebra=auto  EquationFormulation=NE_TIME_EF  DelaysMemoryBudget=1024  AutomaticFiltering=on  FilteringTimeConstant=0.001  PartitionStorageMethod=AS_NEEDED  PartitionMemoryBudget=1024
  Sphere to Plane Force : Contact_Forces_Lib/3D/Sphere to Plane Force  Commented=on  sphere_rad=0.03  plane_lenx=1  plane_leny=1  plane_depth=0.1/2  force_law=Linear  k_contact=1e5  b_contact=1e2  pen_full_damp_F=1e-4  pen_exponent=1  custom_param_1=1  custom_param_2=1  friction_law=Stick-Slip Continuous  mu_kinetic=0.5  mu_static=0.7  v_thr=0.001  vis_on=off  vis_opc_en=0  vis_len_plaBz=0.005  vis_clr=[0.9 0.2 0.2]  vis_opc=0.7
  Transform : sm_lib/Frames and Transforms/Rigid Transform  TranslationMethod=Cartesian  TranslationStandardOffset=0  TranslationLengthUnit=mm  TranslationStandardAxis=+Z  TranslationCartesianOffset=smiData.RigidTransform(9).translation  TranslationROffset=0  TranslationROffsetUnits=m  TranslationZOffset=0  TranslationZOffsetUnits=m  TranslationThetaOffset=0  TranslationThetaOffsetUnits=deg  RotationMethod=ArbitraryAxis  RotationAngleUnits=rad  RotationStandardAxis=+Z  RotationAngle=smiData.RigidTransform(9).angle  RotationArbitraryAxis=smiData.RigidTransform(9).axis  FollAlignAxisA=+X  BaseAlignAxisA=+Y  FollAlignAxisB=+Y  BaseAlignAxisB=+Z  RotationSequenceAxes=FollowerAxes  RotationSequence=XYX  RotationSequenceAngles=[0 0 0]  RotationSequenceAnglesUnits=deg  RotationMatrix=[1 0 0; 0 1 0; 0 0 1]
  Transform Sensor : sm_lib/Frames and Transforms/Transform Sensor  MeasurementFrame=World  SenseAngle=off  SenseAxis=off  SenseAngle1=off  SenseAngle2=off  SenseAngle3=off  SenseQ=off  SenseR=off  SenseOmegaX=off  SenseOmegaY=off  SenseOmegaZ=off  SenseOmega1=off  SenseOmega2=off  SenseOmega3=off  SenseQDot=off  SenseRDot=off  SenseAlphaX=off  SenseAlphaY=off  SenseAlphaZ=off  SenseAlpha1=off  SenseAlpha2=off  SenseAlpha3=off  SenseQDDot=off  SenseRDDot=off  SenseX=off  SenseY=off  SenseZ=on  SenseRad=off  SenseAzim=off  SenseDist=off  SenseInc=off  SenseXDot=on  SenseYDot=on  SenseZDot=on  SenseRadDot=off  SenseAzimDot=off  SenseDistDot=off  SenseIncDot=off  SenseXDDot=off  SenseYDDot=off  SenseZDDot=off  SenseRadDDot=off  SenseAzimDDot=off  SenseDistDDot=off  SenseIncDDot=off
  World : sm_lib/Frames and Transforms/World Frame
  contact Force : Subsystem
  weld_{1..4} (4 alike) : sm_lib/Joints/Weld Joint  SenseConstraintForce=off  SenseConstraintForceX=off  SenseConstraintForceY=off  SenseConstraintForceZ=off  SenseConstraintTorque=off  SenseConstraintTorqueX=off  SenseConstraintTorqueY=off  SenseConstraintTorqueZ=off  SenseTotalForce=off  SenseTotalForceX=off  SenseTotalForceY=off  SenseTotalForceZ=off  SenseTotalTorque=off  SenseTotalTorqueX=off  SenseTotalTorqueY=off  SenseTotalTorqueZ=off  CompositeWrenchDir=FollowerOnBase  CompositeWrenchFrame=BaseFrame
  q : Outport
  dq : Outport  Port=2
  torque : Outport  Port=3
  Fe1 : Outport  Port=4
  wires:
  Demux/4 -> Simulink-PS Converter3/1
  Mux1/1 -> dq/1
  PS-Simulink Converter10/1 -> Mux2/3
  PS-Simulink Converter8/1 -> Mux2/1
  Demux/1 -> Simulink-PS Converter/1
  PS-Simulink Converter11/1 -> Mux2/4
  PS-Simulink Converter5/1 -> Mux1/2
  PS-Simulink Converter/1 -> Mux/1
  Mux2/1 -> torque/1
  PS-Simulink Converter1/1 -> Mux/2
  Demux/2 -> Simulink-PS Converter1/1
  PS-Simulink Converter9/1 -> Mux2/2
  PS-Simulink Converter6/1 -> Mux1/3
  PS-Simulink Converter7/1 -> Mux1/4
  PS-Simulink Converter4/1 -> Mux1/1
  Mux/1 -> q/1
  PS-Simulink Converter2/1 -> Mux/3
  PS-Simulink Converter3/1 -> Mux/4
  Mux3/1 -> Get Transform/1
  Constant/1 -> Mux3/1
  Constant1/1 -> Mux3/2
  Constant2/1 -> Mux3/3
  Constant3/1 -> Mux3/4
  u/1 -> Demux/1
  Get Transform/1 -> Display/1
  Constant4/1 -> Mux4/1
  Constant5/1 -> Mux4/3, Mux4/2
  PS-Simulink Converter29/1 -> Scope/1, contact Force/1(pZ)
  PS-Simulink Converter12/1 -> contact Force/2(vZ)
  PS-Simulink Converter14/1 -> contact Force/4(vY)
  PS-Simulink Converter13/1 -> contact Force/3(vX)
  Demux/3 -> Simulink-PS Converter2/1
  Sphere to Plane Force/1 -> Bus Selector/1
  Bus Selector/1 -> Mux4/6  "<Normal Force>"
  Bus Selector/2 -> Demux1/1  "<Friction Force>"
  Demux1/2 -> Mux4/5
  Demux1/1 -> Mux4/4, Scope1/1
  Constant8/1 -> Mux5/3, Mux5/2
  Constant6/1 -> Mux5/1
  Signal Builder1/1(Signal 1) -> Gain/1
  contact Force/2(Fx) -> Simulink-PS Converter4/1
  contact Force/3(Fy) -> Simulink-PS Converter5/1
  contact Force/4(Fz) -> Simulink-PS Converter6/1
  Gain/1 -> Mux5/4, Simulink-PS Converter7/1
  Constant7/1 -> Mux5/6, Mux5/5
  contact Force/1(Force) -> Fe1/1
  connections:
  Revolute2/RConn3 -- PS-Simulink Converter7/LConn1
  Revolute/RConn2 -- PS-Simulink Converter1/LConn1
  Link2_1_RIGID/LConn1 -- Revolute/RConn1
  Move_1_RIGID/LConn1 -- Prismatic/RConn1
  Link1_1_RIGID/LConn1 -- Revolute1/RConn1
  Base_1_RIGID/LConn1 -- Transform/RConn1
  Revolute2/RConn2 -- PS-Simulink Converter3/LConn1
  Revolute1/LConn2 -- Simulink-PS Converter/RConn1
  Revolute1/RConn3 -- PS-Simulink Converter4/LConn1
  Simulink-PS Converter3/RConn1 -- Revolute2/LConn2
  Revolute1/RConn4 -- PS-Simulink Converter8/LConn1
  Move_1_RIGID/RConn1 -- Revolute2/LConn1
  PS-Simulink Converter/LConn1 -- Revolute1/RConn2
  Revolute/RConn4 -- PS-Simulink Converter9/LConn1
  Link2_1_RIGID/RConn1 -- Prismatic/LConn1
  Base_1_RIGID/RConn1 -- Revolute1/LConn1
  Link1_1_RIGID/RConn1 -- Revolute/LConn1
  Revolute2/RConn1 -- Rot_1_RIGID/LConn1
  Prismatic/RConn2 -- PS-Simulink Converter2/LConn1
  Revolute2/RConn4 -- PS-Simulink Converter11/LConn1
  Simulink-PS Converter2/RConn1 -- Prismatic/LConn2
  Simulink-PS Converter1/RConn1 -- Revolute/LConn2
  Revolute/RConn3 -- PS-Simulink Converter5/LConn1
  Prismatic/RConn3 -- PS-Simulink Converter6/LConn1
  Rot_1_RIGID/RConn1 -- weld_2/LConn1
  EndEff/LConn1 -- weld_2/RConn1 -- weld_3/LConn1
  Origin/LConn1 -- weld_1/RConn1
  weld_3/RConn1 -- External Force and Torque SphF/RConn1 -- Sphere to Plane Force/LConn1 -- External Force and Torque SphF1/RConn1 -- Ball/LConn1 -- Transform Sensor/RConn1
  PS-Simulink Converter29/LConn1 -- Transform Sensor/RConn2
  weld_4/RConn1 -- Planar Object/LConn1
  PS-Simulink Converter10/LConn1 -- Prismatic/RConn4
  Transform Sensor/RConn3 -- PS-Simulink Converter13/LConn1
  Transform Sensor/RConn4 -- PS-Simulink Converter14/LConn1
  Transform Sensor/RConn5 -- PS-Simulink Converter12/LConn1
  Sphere to Plane Force/RConn1 -- Planar Object/LConn2
  Simulink-PS Converter4/RConn1 -- External Force and Torque SphF/LConn1
  Simulink-PS Converter5/RConn1 -- External Force and Torque SphF/LConn2
  Simulink-PS Converter6/RConn1 -- External Force and Torque SphF/LConn3
  Simulink-PS Converter7/RConn1 -- External Force and Torque SphF1/LConn1
  MechanismConfiguration/RConn1 -- weld_1/LConn1 -- Transform/LConn1 -- weld_4/LConn1 -- Transform Sensor/LConn1 -- Solver Configuration/RConn1 -- World/RConn1

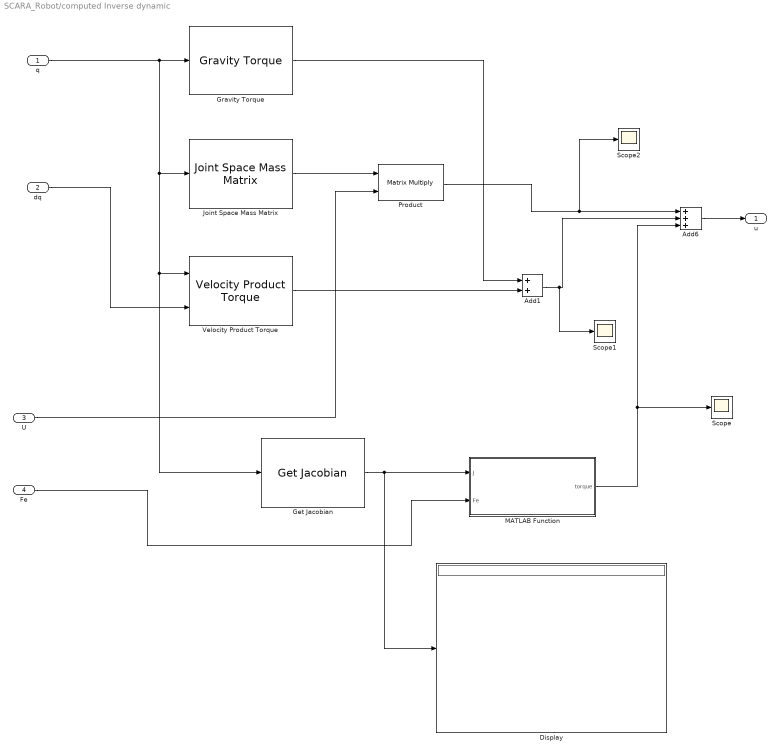
== system SCARA_Robot/computed Inverse dynamic ==
  q : Inport
  dq : Inport  Port=2
  U : Inport  Port=3
  Fe : Inport  Port=4
  Add1 : Sum
  Add6 : Sum  Inputs=+++
  Display : Display
  Get Jacobian : robotmaniplib/Get Jacobian  RigidBodyTree=SCARA_Robot  EndEffector=Body5
      settings: SourceProductName=Robotics System Toolbox
  Gravity Torque : robotmaniplib/Gravity Torque  RigidBodyTree=SCARA_Robot
      settings: SourceProductName=Robotics System Toolbox
  Joint Space Mass Matrix : robotmaniplib/Joint Space Mass Matrix  RigidBodyTree=SCARA_Robot
      settings: SourceProductName=Robotics System Toolbox
  MATLAB Function : MATLAB Function  TreatAsAtomicUnit=on
  Product : Product  Multiplication=Matrix(*)
  Scope : Scope
  Scope1 : Scope
  Scope2 : Scope
  Velocity Product Torque : robotmaniplib/Velocity Product Torque  RigidBodyTree=SCARA_Robot
      settings: SourceProductName=Robotics System Toolbox
  u : Outport
  wires:
  q/1 -> Get Jacobian/1, Velocity Product Torque/1, Joint Space Mass Matrix/1, Gravity Torque/1
  dq/1 -> Velocity Product Torque/2
  Gravity Torque/1 -> Add1/1
  Joint Space Mass Matrix/1 -> Product/1
  Velocity Product Torque/1 -> Add1/2
  Add1/1 -> Scope1/1, Add6/2
  Product/1 -> Scope2/1, Add6/1
  Add6/1 -> u/1
  U/1 -> Product/2
  Get Jacobian/1 -> Display/1, MATLAB Function/1(J)
  Fe/1 -> MATLAB Function/2(Fe)
  MATLAB Function/1(torque) -> Scope/1, Add6/3

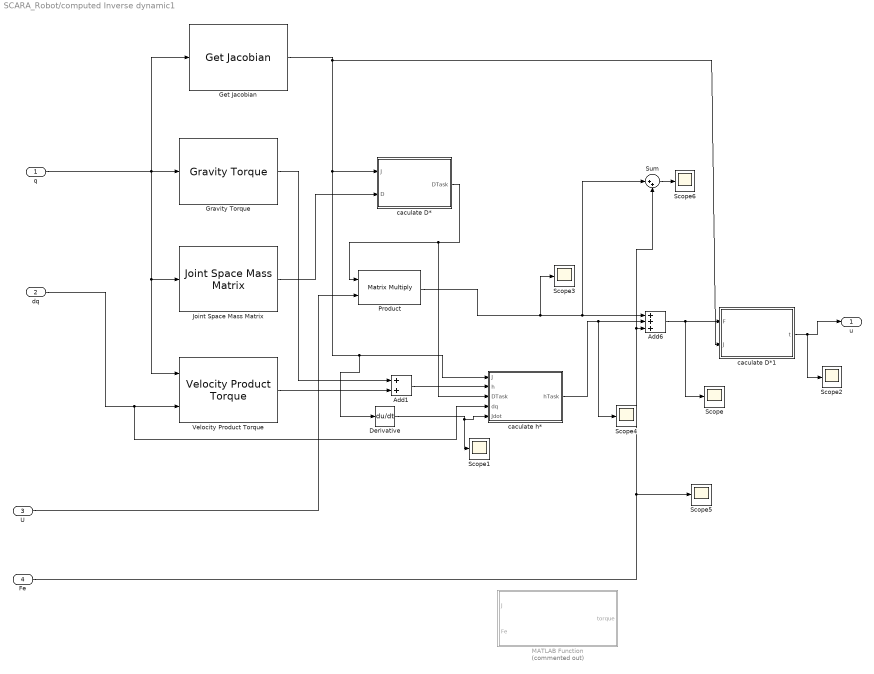
== system SCARA_Robot/computed Inverse dynamic1 ==
  q : Inport
  dq : Inport  Port=2
  U : Inport  Port=3
  Fe : Inport  Port=4
  Add1 : Sum
  Add6 : Sum  Inputs=+++
  Derivative : Derivative
  Get Jacobian : robotmaniplib/Get Jacobian  RigidBodyTree=SCARA_Robot  EndEffector=Body5
      settings: SourceProductName=Robotics System Toolbox
  Gravity Torque : robotmaniplib/Gravity Torque  RigidBodyTree=SCARA_Robot
      settings: SourceProductName=Robotics System Toolbox
  Joint Space Mass Matrix : robotmaniplib/Joint Space Mass Matrix  RigidBodyTree=SCARA_Robot
      settings: SourceProductName=Robotics System Toolbox
  MATLAB Function : MATLAB Function  Commented=on  TreatAsAtomicUnit=on
  Product : Product  Multiplication=Matrix(*)
  Scope{,1..6} (7 alike) : Scope
  Sum : Sum  Inputs=|++
  Velocity Product Torque : robotmaniplib/Velocity Product Torque  RigidBodyTree=SCARA_Robot
      settings: SourceProductName=Robotics System Toolbox
  caculate D* : MATLAB Function  TreatAsAtomicUnit=on
  caculate D*1 : MATLAB Function  TreatAsAtomicUnit=on
  caculate h* : MATLAB Function  TreatAsAtomicUnit=on
  u : Outport
  wires:
  q/1 -> Velocity Product Torque/1, Joint Space Mass Matrix/1, Get Jacobian/1, Gravity Torque/1
  Velocity Product Torque/1 -> Add1/2
  U/1 -> Product/2
  Joint Space Mass Matrix/1 -> caculate D*/2(D)
  Get Jacobian/1 -> Derivative/1, caculate h*/1(J), caculate D*/1(J), caculate D*1/2(J)
  caculate D*/1(DTask) -> caculate h*/3(DTask), Product/1
  Product/1 -> Scope3/1, Sum/1, Add6/1
  Fe/1 -> Scope5/1, Sum/2, Add6/3
  Gravity Torque/1 -> Add1/1
  Add1/1 -> caculate h*/2(h)
  dq/1 -> caculate h*/4(dq), Velocity Product Torque/2
  caculate D*1/1(t) -> Scope2/1, u/1
  Add6/1 -> Scope/1, caculate D*1/1(F)
  Derivative/1 -> Scope1/1, caculate h*/5(Jdot)
  caculate h*/1(hTask) -> Scope4/1, Add6/2
  Sum/1 -> Scope6/1

== system SCARA_Robot/SimscapeModelwithContactModel/Base_1_RIGID ==
  ReferenceFrame : sm_lib/Frames and Transforms/Reference Frame
  Solid : sm_lib/Body Elements/Solid  InertiaType=Custom  Mass=smiData.Solid(3).mass  MassUnits=kg  CenterOfMass=smiData.Solid(3).CoM  CenterOfMassUnits=mm  MomentsOfInertia=smiData.Solid(3).MoI  MomentsOfInertiaUnits=kg*mm^2  ProductsOfInertia=smiData.Solid(3).PoI  ProductsOfInertiaUnits=kg*mm^2  BasedOnType=Density  Density=1000  DensityUnits=kg/m^3  DoExposeReferenceFrame=off  SerializedFrames=<Frames><Frame><Id>Frame1</Id><Value><Name>F2</Name><Origin><Source>GeometricFeature</Source><FeatureName>cylindrical surface 2</FeatureName></Origin><PrimaryAxis><DefinedDirection>+Z</DefinedDirection><Source>ReferenceFrame</Source><SourceDirection>+Z</SourceDirection><FeatureName></FeatureName></PrimaryAxis><SecondaryAxis><DefinedDirection>+X</DefinedDirection><Source>ReferenceFrame</Source><SourceDirection>+X</SourceDirection><FeatureName></FeatureName></SecondaryAxis></Value></Frame></Frames>  GraphicType=FromGeometry  MarkerShape=Sphere  MarkerSize=10  GraphicVisPropType=SimpleVisualProperties  GraphicDiffuseColor=smiData.Solid(3).color  GraphicSpecularColor=[0.5 0.5 0.5 1.0]  GraphicAmbientColor=[0.15 0.15 0.15 1.0]  GraphicEmissiveColor=[0.0 0.0 0.0 1.0]  GraphicShininess=75  GraphicOpacity=smiData.Solid(3).opacity  GeometryShape=FromFile  RectangleSize=[1 1]  RectangleSizeUnits=m  BrickDimensions=[1 1 1]  BrickDimensionUnits=m  CylinderRadius=1  CylinderRadiusUnits=m  CylinderLength=1  CylinderLengthUnits=m  SphereRadius=1  SphereRadiusUnits=m  EllipsoidRadii=[1 1 1]  EllipsoidRadiiUnits=m  ExtrusionCrossSection=[1 1; -1 1; -1 -1; 1 -1]  ExtrusionCrossSectionUnits=m  ExtrusionLength=1  ExtrusionLengthUnits=m  PolygonNumSides=3  PolygonOuterRadius=1  PolygonOuterRadiusUnits=m  ExtGeomFileType=STEP  ExtGeomFileName=Base_默认_sldprt.STEP  ExtGeomFileUnits=m  RevolutionCrossSection=[1 1; 1 -1; 2 -1; 2 1]  RevolutionCrossSectionUnits=m  RevolutionExtent=Full  RevolutionAngle=180  RevolutionAngleUnits=deg
  Transform : sm_lib/Frames and Transforms/Rigid Transform  TranslationMethod=Cartesian  TranslationStandardOffset=0  TranslationLengthUnit=mm  TranslationStandardAxis=+Z  TranslationCartesianOffset=smiData.RigidTransform(3).translation  TranslationROffset=0  TranslationROffsetUnits=m  TranslationZOffset=0  TranslationZOffsetUnits=m  TranslationThetaOffset=0  TranslationThetaOffsetUnits=deg  RotationMethod=ArbitraryAxis  RotationAngleUnits=rad  RotationStandardAxis=+Z  RotationAngle=smiData.RigidTransform(3).angle  RotationArbitraryAxis=smiData.RigidTransform(3).axis  FollAlignAxisA=+X  BaseAlignAxisA=+Y  FollAlignAxisB=+Y  BaseAlignAxisB=+Z  RotationSequenceAxes=FollowerAxes  RotationSequence=XYX  RotationSequenceAngles=[0 0 0]  RotationSequenceAnglesUnits=deg  RotationMatrix=[1 0 0; 0 1 0; 0 0 1]
  F1 : PMIOPort  Side=Left
  F : PMIOPort  Port=2  Side=Right
  connections:
  ReferenceFrame/RConn1 -- Solid/LConn1 -- Transform/LConn1 -- F1/RConn1
  Transform/RConn1 -- F/RConn1

== system SCARA_Robot/SimscapeModelwithContactModel/Contact Force1 ==
  Planar Object : Subsystem
  Sphere to Plane Force : Contact_Forces_Lib/3D/Sphere to Plane Force  sphere_rad=Ball.radius  plane_lenx=Plane.width  plane_leny=Plane.length  plane_depth=0.1/2  force_law=Nonlinear  k_contact=1e7  b_contact=1e3  pen_full_damp_F=1e-4  pen_exponent=1  custom_param_1=1  custom_param_2=1  friction_law=None  mu_kinetic=0.5  mu_static=0.7  v_thr=0.001  vis_on=off  vis_opc_en=0  vis_len_plaBz=Plane.depth*0.1  vis_clr=[0.9 0.2 0.2]  vis_opc=0.7
  weld_3 : sm_lib/Joints/Weld Joint  SenseConstraintForce=off  SenseConstraintForceX=off  SenseConstraintForceY=off  SenseConstraintForceZ=off  SenseConstraintTorque=off  SenseConstraintTorqueX=off  SenseConstraintTorqueY=off  SenseConstraintTorqueZ=off  SenseTotalForce=off  SenseTotalForceX=off  SenseTotalForceY=off  SenseTotalForceZ=off  SenseTotalTorque=off  SenseTotalTorqueX=off  SenseTotalTorqueY=off  SenseTotalTorqueZ=off  CompositeWrenchDir=FollowerOnBase  CompositeWrenchFrame=BaseFrame
  SphFace : PMIOPort  Side=Left
  plate : PMIOPort  Port=2  Side=Left
  Force : Outport
  wires:
  Sphere to Plane Force/1 -> Force/1  "Sph2Pl_bus"
  connections:
  weld_3/RConn1 -- Planar Object/LConn1
  SphFace/RConn1 -- Sphere to Plane Force/LConn1
  weld_3/LConn1 -- plate/RConn1
  Planar Object/LConn2 -- Sphere to Plane Force/RConn1

== system SCARA_Robot/SimscapeModelwithContactModel/EndEff ==
  ReferenceFrame : sm_lib/Frames and Transforms/Reference Frame
  F : PMIOPort  Side=Left
  connections:
  ReferenceFrame/RConn1 -- F/RConn1
